simulink library "aoc"  (Simulink 8.1)
settings: Solver=ode45  StartTime=0.0  StopTime=10.0  RelTol=1e-3
settings Model: Creator=AT015086  LastModifiedBy=tescamilla

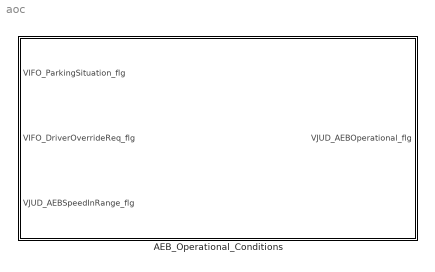
== system aoc ==
  AEB_Operational_Conditions : Subsystem

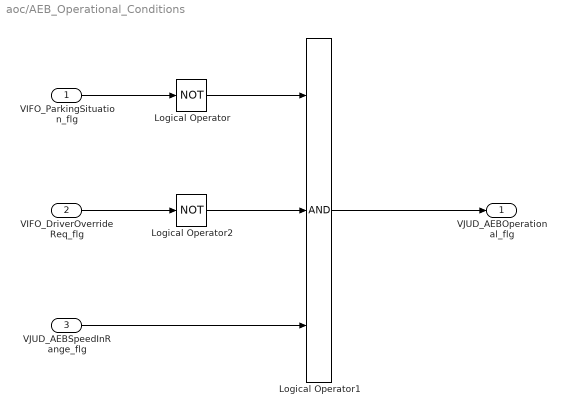
== system aoc/AEB_Operational_Conditions ==
  VIFO_ParkingSituation_flg : Inport
  VIFO_DriverOverrideReq_flg : Inport  Port=2
  VJUD_AEBSpeedInRange_flg : Inport  Port=3
  Logical Operator : Logic  Operator=NOT  AllPortsSameDT=off  OutDataTypeStr=boolean
  Logical Operator1 : Logic  Inputs=3  AllPortsSameDT=off  OutDataTypeStr=boolean
  Logical Operator2 : Logic  Operator=NOT  AllPortsSameDT=off  OutDataTypeStr=boolean
  VJUD_AEBOperational_flg : Outport
  wires:
  VJUD_AEBSpeedInRange_flg/1 -> Logical Operator1/3
  Logical Operator1/1 -> VJUD_AEBOperational_flg/1
  VIFO_ParkingSituation_flg/1 -> Logical Operator/1
  VIFO_DriverOverrideReq_flg/1 -> Logical Operator2/1
  Logical Operator2/1 -> Logical Operator1/2
  Logical Operator/1 -> Logical Operator1/1
